simulink model "Team37_Quadcopter_Simulation"  (R2013b)
settings: Solver=ode45  StartTime=0  StopTime=5  FixedStep=0.005  RelTol=1e-3
model workspace (MAT data in the model file):
  MCOS : class17 (value not decoded)
undefined symbols (not defined in the file): DiscIntNeverNeededParam, IC, quadModel
libraries: simulink x8
(part 2 of 2)

== system Team37_Quadcopter_Simulation/On-board State Estimation/filterRawData()/Filter IC fixer ==
  FilterStart : Inport
  Normal Output : Inport  Port=2
  Constant : Constant
  IC : InitialCondition  Value=0
  Switch : Switch  Criteria=u2 ~= 0
  Out1 : Outport
  wires:
  Switch/1 -> Out1/1
  FilterStart/1 -> Switch/3
  IC/1 -> Switch/2
  Constant/1 -> IC/1
  Normal Output/1 -> Switch/1

== system Team37_Quadcopter_Simulation/On-board State Estimation/filterRawData()/Filter IC fixer1 ==
  FilterStart : Inport
  Normal Output : Inport  Port=2
  Constant : Constant
  IC : InitialCondition  Value=0
  Switch : Switch  Criteria=u2 ~= 0
  Out1 : Outport
  wires:
  Switch/1 -> Out1/1
  FilterStart/1 -> Switch/3
  IC/1 -> Switch/2
  Constant/1 -> IC/1
  Normal Output/1 -> Switch/1

== system Team37_Quadcopter_Simulation/On-board State Estimation/getMotion6()/Accelerometer ==
  note: NOTE: Change to int16 here!!!
  note: Note: this process is very artificial as it assumes no other acceleration
      | forces act on the body of the vehicle besides gravity, including those from
      | translational motion...
  note: -M sin(The)
  note: M cos(The) sin(Phi)
  note: M cos(Phi) cos(The)
  Phi : Inport
  Theta : Inport  Port=2
  Product : Product
  Product1 : Product
  Raw Data Scaling : Subsystem
  Raw Data Scaling1 : Subsystem
  Raw Data Scaling2 : Subsystem
  Trigonometric Function : Trigonometry  Operator=sincos  OutputSignalType=real
  Trigonometric Function1 : Trigonometry  Operator=sincos  OutputSignalType=real
  ax : Outport
  ay : Outport  Port=2
  az : Outport  Port=3
  wires:
  Phi/1 -> Trigonometric Function/1
  Theta/1 -> Trigonometric Function1/1
  Trigonometric Function/1 -> Product/1  "ax"
  Trigonometric Function1/2 -> Product1/2, Product/2
  Trigonometric Function/2 -> Product1/1
  Raw Data Scaling1/1(Out1) -> ay/1
  Raw Data Scaling2/1(Out1) -> az/1
  Product/1 -> Raw Data Scaling1/1(In1)
  Product1/1 -> Raw Data Scaling2/1(In1)
  Trigonometric Function1/1 -> Raw Data Scaling/1(In1)
  Raw Data Scaling/1(Out1) -> ax/1

== system Team37_Quadcopter_Simulation/On-board State Estimation/getMotion6()/Gyro signals ==
  P : Inport
  Q : Inport  Port=2
  R : Inport  Port=3
  Gyro Raw Data Scaling : Subsystem
  Gyro Raw Data Scaling1 : Subsystem
  Gyro Raw Data Scaling2 : Subsystem
  gx : Outport
  gy : Outport  Port=2
  gz : Outport  Port=3
  wires:
  P/1 -> Gyro Raw Data Scaling/1(In1)
  Q/1 -> Gyro Raw Data Scaling1/1(In1)
  R/1 -> Gyro Raw Data Scaling2/1(In1)
  Gyro Raw Data Scaling/1(Out1) -> gx/1
  Gyro Raw Data Scaling1/1(Out1) -> gy/1
  Gyro Raw Data Scaling2/1(Out1) -> gz/1

== system Team37_Quadcopter_Simulation/Sampled Command Quadcopter Dynamics/Motor Dynamics/Throttle To RPM Gain and Cutoff_1 ==
  note: Output equals linearly scaled RPM
      | for given throttle input if throttle input >=Throttle Cuttoff (minThr)
      | else output is zero.
  In5 : Inport
  Constant : Constant  Value=quadModel.b
  Gain : Gain  Gain=quadModel.cr
  Minimum Throttle Cutoff : simulink/Logic and Bit Operations/Compare To Constant  relop=>=  const=quadModel.minThr  OutDataTypeStr=uint8
  Product : Product
  Sum1 : Sum  Inputs=++|
  Out5 : Outport
  wires:
  Minimum Throttle Cutoff/1 -> Product/2
  Product/1 -> Out5/1
  In5/1 -> Gain/1, Minimum Throttle Cutoff/1
  Gain/1 -> Sum1/2
  Sum1/1 -> Product/1
  Constant/1 -> Sum1/1

== system Team37_Quadcopter_Simulation/Sampled Command Quadcopter Dynamics/Motor Dynamics/Throttle To RPM Gain and Cutoff_2 ==
  note: Output equals linearly scaled RPM
      | for given throttle input if throttle input >=Throttle Cuttoff (minThr)
      | else output is zero.
  In5 : Inport
  Constant : Constant  Value=quadModel.b
  Gain : Gain  Gain=quadModel.cr
  Minimum Throttle Cutoff : simulink/Logic and Bit Operations/Compare To Constant  relop=>=  const=quadModel.minThr  OutDataTypeStr=uint8
  Product : Product
  Sum1 : Sum  Inputs=++|
  Out5 : Outport
  wires:
  Minimum Throttle Cutoff/1 -> Product/2
  Product/1 -> Out5/1
  In5/1 -> Gain/1, Minimum Throttle Cutoff/1
  Gain/1 -> Sum1/2
  Sum1/1 -> Product/1
  Constant/1 -> Sum1/1

== system Team37_Quadcopter_Simulation/Sampled Command Quadcopter Dynamics/Motor Dynamics/Throttle To RPM Gain and Cutoff_3 ==
  note: Output equals linearly scaled RPM
      | for given throttle input if throttle input >=Throttle Cuttoff (minThr)
      | else output is zero.
  In5 : Inport
  Constant : Constant  Value=quadModel.b
  Gain : Gain  Gain=quadModel.cr
  Minimum Throttle Cutoff : simulink/Logic and Bit Operations/Compare To Constant  relop=>=  const=quadModel.minThr  OutDataTypeStr=uint8
  Product : Product
  Sum1 : Sum  Inputs=++|
  Out5 : Outport
  wires:
  Minimum Throttle Cutoff/1 -> Product/2
  Product/1 -> Out5/1
  In5/1 -> Gain/1, Minimum Throttle Cutoff/1
  Gain/1 -> Sum1/2
  Sum1/1 -> Product/1
  Constant/1 -> Sum1/1

== system Team37_Quadcopter_Simulation/Sampled Command Quadcopter Dynamics/Motor Dynamics/Throttle To RPM Gain and Cutoff_4 ==
  note: Output equals linearly scaled RPM
      | for given throttle input if throttle input >=Throttle Cuttoff (minThr)
      | else output is zero.
  In5 : Inport
  Constant : Constant  Value=quadModel.b
  Gain : Gain  Gain=quadModel.cr
  Minimum Throttle Cutoff : simulink/Logic and Bit Operations/Compare To Constant  relop=>=  const=quadModel.minThr  OutDataTypeStr=uint8
  Product : Product
  Sum1 : Sum  Inputs=++|
  Out5 : Outport
  wires:
  Minimum Throttle Cutoff/1 -> Product/2
  Product/1 -> Out5/1
  In5/1 -> Gain/1, Minimum Throttle Cutoff/1
  Gain/1 -> Sum1/2
  Sum1/1 -> Product/1
  Constant/1 -> Sum1/1

== system Team37_Quadcopter_Simulation/On-board State Estimation/State Estimation and Complimentary Mixing/Complimentary Filter/Filter IC fixer ==
  FilterStart : Inport
  Normal Output : Inport  Port=2
  Constant : Constant
  IC : InitialCondition  Value=0
  Switch : Switch  Criteria=u2 ~= 0  SampleTime=ControllerSampleTime
  Out1 : Outport
  wires:
  Switch/1 -> Out1/1
  FilterStart/1 -> Switch/3
  IC/1 -> Switch/2
  Constant/1 -> IC/1
  Normal Output/1 -> Switch/1

== system Team37_Quadcopter_Simulation/On-board State Estimation/State Estimation and Complimentary Mixing/Complimentary Filter/Filter IC fixer1 ==
  FilterStart : Inport
  Normal Output : Inport  Port=2
  Constant : Constant
  IC : InitialCondition  Value=0
  Switch : Switch  Criteria=u2 ~= 0  SampleTime=ControllerSampleTime
  Out1 : Outport
  wires:
  Switch/1 -> Out1/1
  FilterStart/1 -> Switch/3
  IC/1 -> Switch/2
  Constant/1 -> IC/1
  Normal Output/1 -> Switch/1

== system Team37_Quadcopter_Simulation/On-board State Estimation/State Estimation and Complimentary Mixing/Complimentary Filter/Filter IC fixer2 ==
  FilterStart : Inport
  Normal Output : Inport  Port=2
  Constant : Constant
  IC : InitialCondition  Value=0
  Switch : Switch  Criteria=u2 ~= 0  SampleTime=ControllerSampleTime
  Out1 : Outport
  wires:
  Switch/1 -> Out1/1
  FilterStart/1 -> Switch/3
  IC/1 -> Switch/2
  Constant/1 -> IC/1
  Normal Output/1 -> Switch/1

== system Team37_Quadcopter_Simulation/On-board State Estimation/State Estimation and Complimentary Mixing/Subsystem/Filter IC fixer1 ==
  FilterStart : Inport
  Normal Output : Inport  Port=2
  Constant : Constant
  IC : InitialCondition  Value=0
  Switch : Switch  Criteria=u2 ~= 0  SampleTime=ControllerSampleTime
  Out1 : Outport
  wires:
  Switch/1 -> Out1/1
  FilterStart/1 -> Switch/3
  IC/1 -> Switch/2
  Constant/1 -> IC/1
  Normal Output/1 -> Switch/1

== system Team37_Quadcopter_Simulation/On-board State Estimation/State Estimation and Complimentary Mixing/Subsystem/Filter IC fixer2 ==
  FilterStart : Inport
  Normal Output : Inport  Port=2
  Constant : Constant
  IC : InitialCondition  Value=0
  Switch : Switch  Criteria=u2 ~= 0  SampleTime=ControllerSampleTime
  Out1 : Outport
  wires:
  Switch/1 -> Out1/1
  FilterStart/1 -> Switch/3
  IC/1 -> Switch/2
  Constant/1 -> IC/1
  Normal Output/1 -> Switch/1

== system Team37_Quadcopter_Simulation/On-board State Estimation/State Estimation and Complimentary Mixing/Subsystem/Phi_dot composer ==
  note: H_Phi = [1,tan(The)*sin(Phi), tan(The)*cos(Phi);
      |          0,         cos(Phi),         -sin(Phi);
      |          0,sin(Phi)/cos(The),cos(Phi)/cos(The)];
      | Phidot = H_Phi*omb_bi; %% Units OK SI, this is the derivative of the Euler angles
  Phi : Inport
  Theta : Inport  Port=2
  P : Inport  Port=3
  Q : Inport  Port=4
  R : Inport  Port=5
  Product : Product  Inputs=3
  Product1 : Product  Inputs=3
  Sum : Sum  Inputs=+++
  Trigonometric Function : Trigonometry  Operator=tan
  Trigonometric Function1 : Trigonometry  Operator=sincos
  phiDot : Outport
  wires:
  Sum/1 -> phiDot/1
  Trigonometric Function/1 -> Product1/1, Product/1
  Product1/1 -> Sum/3
  Q/1 -> Product/3
  Trigonometric Function1/1 -> Product/2
  Phi/1 -> Trigonometric Function1/1
  Theta/1 -> Trigonometric Function/1
  P/1 -> Sum/1
  R/1 -> Product1/3
  Product/1 -> Sum/2
  Trigonometric Function1/2 -> Product1/2

== system Team37_Quadcopter_Simulation/On-board State Estimation/State Estimation and Complimentary Mixing/Subsystem/Phi_dot composer1 ==
  note: H_Phi = [1,tan(The)*sin(Phi), tan(The)*cos(Phi);
      |          0,         cos(Phi),         -sin(Phi);
      |          0,sin(Phi)/cos(The),cos(Phi)/cos(The)];
      | Phidot = H_Phi*omb_bi; %% Units OK SI
  Phi : Inport
  Theta : Inport  Port=2
  Q : Inport  Port=3
  R : Inport  Port=4
  Divide : Product  Inputs=**/
  Divide1 : Product  Inputs=**/
  Sum : Sum  Inputs=|++
  Trigonometric Function : Trigonometry  Operator=sincos
  Trigonometric Function1 : Trigonometry  Operator=cos
  psiDot : Outport
  wires:
  Sum/1 -> psiDot/1
  Phi/1 -> Trigonometric Function/1
  Trigonometric Function/1 -> Divide/2
  Theta/1 -> Trigonometric Function1/1
  Divide/1 -> Sum/1
  Trigonometric Function1/1 -> Divide/3, Divide1/3
  Q/1 -> Divide/1
  R/1 -> Divide1/2
  Divide1/1 -> Sum/2
  Trigonometric Function/2 -> Divide1/1

== system Team37_Quadcopter_Simulation/On-board State Estimation/State Estimation and Complimentary Mixing/Subsystem/Theta_dot composer1 ==
  note: H_Phi = [1,tan(The)*sin(Phi), tan(The)*cos(Phi);
      |          0,         cos(Phi),         -sin(Phi);
      |          0,sin(Phi)/cos(The),cos(Phi)/cos(The)];
      | Phidot = H_Phi*omb_bi; %% Units OK SI
  Phi : Inport
  Q : Inport  Port=2
  R : Inport  Port=3
  Product : Product
  Product1 : Product
  Scope : Scope  NumInputPorts=2
      settings: YMin=-5~-5  YMax=5~5  SaveName=ScopeData6
  Sum : Sum  Inputs=|++
  Trigonometric Function2 : Trigonometry  Operator=sincos
  Unary Minus : UnaryMinus
  thetaDot : Outport
  wires:
  Sum/1 -> thetaDot/1
  Phi/1 -> Trigonometric Function2/1
  Q/1 -> Product/2
  Product/1 -> Sum/1
  Trigonometric Function2/1 -> Scope/2, Unary Minus/1
  Unary Minus/1 -> Scope/1, Product1/1
  R/1 -> Product1/2
  Product1/1 -> Sum/2
  Trigonometric Function2/2 -> Product/1

== system Team37_Quadcopter_Simulation/On-board State Estimation/State Estimation and Complimentary Mixing/Subsystem1/Magnitude ==
  x_acc : Inport
  y_acc : Inport  Port=2
  z_acc : Inport  Port=3
  Demux1 : Demux  Outputs=3
  Math Function : Math  Operator=square  SaturateOnIntegerOverflow=on
  Mux : Mux  Inputs=3
  Sqrt : Sqrt  SaturateOnIntegerOverflow=on
  Sum : Sum  Inputs=+++
  |g| : Outport
  wires:
  Sqrt/1 -> |g|/1  "mag_acc"
  Sum/1 -> Sqrt/1
  Demux1/3 -> Sum/3
  Mux/1 -> Math Function/1
  Math Function/1 -> Demux1/1
  Demux1/1 -> Sum/1
  Demux1/2 -> Sum/2
  y_acc/1 -> Mux/2
  x_acc/1 -> Mux/1
  z_acc/1 -> Mux/3

== system Team37_Quadcopter_Simulation/On-board State Estimation/getMotion6()/Accelerometer/Raw Data Scaling ==
  In1 : Inport
  Data Type Conversion : DataTypeConversion  OutDataTypeStr=int16  SaturateOnIntegerOverflow=on
  Gain1 : Gain  Gain=-16384  RndMeth=Round  SaturateOnIntegerOverflow=on
  Out1 : Outport
  wires:
  Gain1/1 -> Data Type Conversion/1
  In1/1 -> Gain1/1
  Data Type Conversion/1 -> Out1/1

== system Team37_Quadcopter_Simulation/On-board State Estimation/getMotion6()/Accelerometer/Raw Data Scaling1 ==
  In1 : Inport
  Data Type Conversion : DataTypeConversion  OutDataTypeStr=int16
  Gain1 : Gain  Gain=16384  RndMeth=Round  SaturateOnIntegerOverflow=on
  Out1 : Outport
  wires:
  Gain1/1 -> Data Type Conversion/1
  In1/1 -> Gain1/1
  Data Type Conversion/1 -> Out1/1

== system Team37_Quadcopter_Simulation/On-board State Estimation/getMotion6()/Accelerometer/Raw Data Scaling2 ==
  In1 : Inport
  Data Type Conversion : DataTypeConversion  OutDataTypeStr=int16
  Gain1 : Gain  Gain=16384  RndMeth=Round  SaturateOnIntegerOverflow=on
  Out1 : Outport
  wires:
  Gain1/1 -> Data Type Conversion/1
  In1/1 -> Gain1/1
  Data Type Conversion/1 -> Out1/1

== system Team37_Quadcopter_Simulation/On-board State Estimation/getMotion6()/Gyro signals/Gyro Raw Data Scaling ==
  In1 : Inport
  Data Type Conversion : DataTypeConversion  OutDataTypeStr=int16  SaturateOnIntegerOverflow=on
  Gain1 : Gain  Gain=180*131.1/pi  RndMeth=Round  SaturateOnIntegerOverflow=on
  Out1 : Outport
  wires:
  Gain1/1 -> Data Type Conversion/1
  In1/1 -> Gain1/1
  Data Type Conversion/1 -> Out1/1

== system Team37_Quadcopter_Simulation/On-board State Estimation/getMotion6()/Gyro signals/Gyro Raw Data Scaling1 ==
  In1 : Inport
  Data Type Conversion : DataTypeConversion  OutDataTypeStr=int16  SaturateOnIntegerOverflow=on
  Gain1 : Gain  Gain=180*131.1/pi  RndMeth=Round  SaturateOnIntegerOverflow=on
  Out1 : Outport
  wires:
  Gain1/1 -> Data Type Conversion/1
  In1/1 -> Gain1/1
  Data Type Conversion/1 -> Out1/1

== system Team37_Quadcopter_Simulation/On-board State Estimation/getMotion6()/Gyro signals/Gyro Raw Data Scaling2 ==
  In1 : Inport
  Data Type Conversion : DataTypeConversion  OutDataTypeStr=int16  SaturateOnIntegerOverflow=on
  Gain1 : Gain  Gain=180*131.1/pi  RndMeth=Round  SaturateOnIntegerOverflow=on
  Out1 : Outport
  wires:
  Gain1/1 -> Data Type Conversion/1
  In1/1 -> Gain1/1
  Data Type Conversion/1 -> Out1/1
